simulink model "d_tanh_test"  (R2022a)
settings: Solver=VariableStepAuto  StartTime=0.0  StopTime=3000  RelTol=1e-3
libraries: dspsrcs4 x1, modelsimlib x1
settings Model: Creator=jose_  LastModifiedBy=jose_

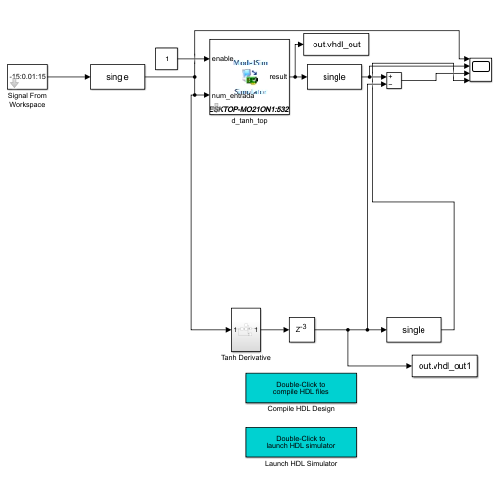
[thumbnail: Simulink's stored preview of the top-level diagram]
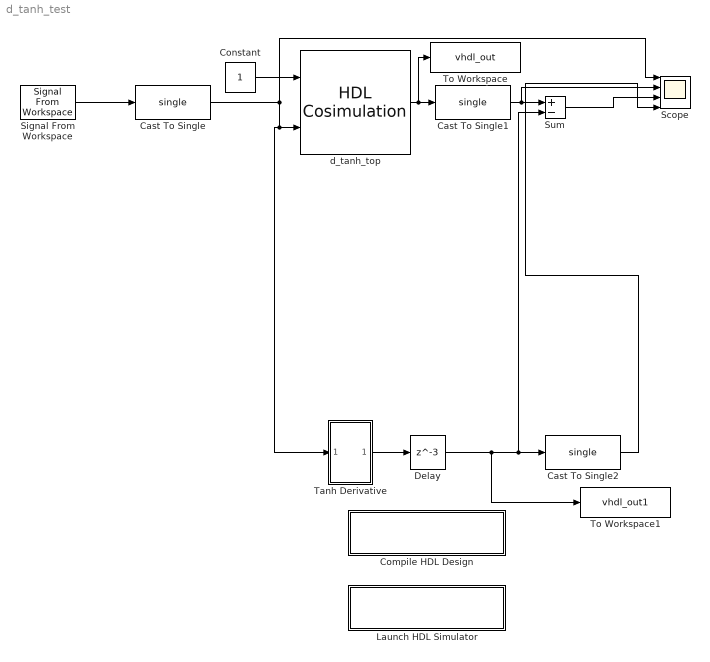
== system d_tanh_test ==
  Cast To Single : DataTypeConversion  OutDataTypeStr=single  SaturateOnIntegerOverflow=off  RndMeth=Floor
  Cast To Single1 : DataTypeConversion  OutDataTypeStr=single  SaturateOnIntegerOverflow=off  RndMeth=Floor
  Cast To Single2 : DataTypeConversion  OutDataTypeStr=single  SaturateOnIntegerOverflow=off  RndMeth=Floor
  Compile HDL Design : Subsystem
      settings: OpenFcn=eval('compile_hdl_design_d_tanh_top');
      mask Display: disp(['Double-Click to' char(10) 'compile HDL files'])
  Constant : Constant  OutDataTypeStr=fixdt(0,1,0)
  Delay : Delay  DelayLength=3
  Launch HDL Simulator : Subsystem
      settings: OpenFcn=eval('launch_hdl_simulator_d_tanh_top');
      mask Display: disp(['Double-Click to' char(10) 'launch HDL simulator'])
  Scope : Scope  NumInputPorts=4
  Signal From Workspace : dspsrcs4/Signal From Workspace  X=-15:0.01:15  Ts=1  nsamps=1  OutputAfterFinalValue=Setting to zero  ignoreOrWarnInputAndFrameLengths=off  OutputFrames=off
  Sum : Sum  Inputs=|+|-|
  Tanh Derivative : Subsystem
  To Workspace : ToWorkspace  VariableName=vhdl_out  SampleTime=-1
      settings: Save2DSignal=2-D array (concatenate along first dimension)
  To Workspace1 : ToWorkspace  VariableName=vhdl_out1  SampleTime=-1
      settings: Save2DSignal=2-D array (concatenate along first dimension)
  d_tanh_top : modelsimlib/HDL Cosimulation  PortPaths=/d_tanh_top/enable;/d_tanh_top/num_entrada;/d_tanh_top/result  PortModes=[1 1 2 ]  PortTimes=[-1,-1,1]  PortSigns=[-1 -1 3 ]  PortFracLengths=[0,0,0]  CommLocal=on  CommSharedMemory=off  CommPortNumber=53203  CommShowInfo=on  ClockModes=[]  ClockTimes=[]  TclPreSimCommand=|  TclPostSimCommand=|  TimingMode=ns  TimingScaleFactor=20  idxCellArray={'UNUSED_VAR'}  CosimBypass=Full Simulation  AllowDirectFeedthrough=on  ProductName=EDA Simulator Link MQ  RunAutoTimescale=off  HdlClocks=/d_tanh_top/clk 20 ns;  PreRunTime=20  PreRunTimeUnit=ns
      TclPreSimCommand=|
      | force /d_tanh_top/clk 0 0 ns, 1 10 ns -repeat 20 ns;
      | force /d_tanh_top/rst 0 0 ns, 1 8 ns;
      TclPostSimCommand=|
      | noforce /d_tanh_top/clk;
      | noforce /d_tanh_top/rst;
      | puts "done";
      settings: SourceProductBaseCode=ES
  wires:
  Signal From Workspace/1 -> Cast To Single/1
  Cast To Single/1 -> d_tanh_top/2, Tanh Derivative/1(In1), Scope/1
  Tanh Derivative/1(Out1) -> Delay/1
  Delay/1 -> To Workspace1/1, Cast To Single2/1, Sum/2
  Sum/1 -> Scope/3
  Constant/1 -> d_tanh_top/1
  d_tanh_top/1 -> To Workspace/1, Cast To Single1/1
  Cast To Single1/1 -> Scope/2, Sum/1
  Cast To Single2/1 -> Scope/4

== system d_tanh_test/Compile HDL Design ==

== system d_tanh_test/Launch HDL Simulator ==

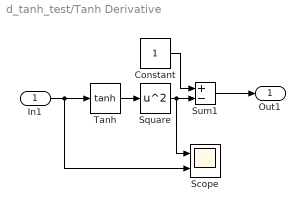
== system d_tanh_test/Tanh Derivative ==
  In1 : Inport
  Constant : Constant
  Scope : Scope  NumInputPorts=2
  Square : Math  Operator=square  OutputSignalType=real
  Sum1 : Sum  Inputs=|+|-|
  Tanh : Trigonometry  Operator=tanh  OutputSignalType=real
  Out1 : Outport
  wires:
  In1/1 -> Scope/2, Tanh/1
  Sum1/1 -> Out1/1
  Tanh/1 -> Square/1
  Constant/1 -> Sum1/1
  Square/1 -> Scope/1, Sum1/2
